simulink model "PubIfDecisionTOS_MDL"  (R2020b)
settings: configuration reference "DspaceConfig" (kept outside this file)
PostLoadFcn:
  | if any(exist('dsrtsu_mdlpostloadfcn', 'file') ~= 0), dsrtsu_mdlpostloadfcn('Execute', bdroot); end
InitFcn:
  | , if any(exist('dsmpb_private', 'file') ~= 0), dsmpb_private('dsmpb_mdlclblib', 'Init', bdroot); end,
undefined symbols (not defined in the file or in its folder): C_TOS_ACCEgoRAxletoFbumplength_m, C_TOS_ACCTargetFront_Flag, C_TOS_AEBJAPedObjDxThre_Val, C_TOS_AEBJAPedObjDyThre_Val, C_TOS_AEBJATargetSize_Val, C_TOS_AEBJAVehObjDxThre_Val, C_TOS_AEBJAVehObjDyThre_Val, C_TOS_AEBJuncPedTargetSize_Val, C_TOS_AEBLatObjDxThre_Val, C_TOS_AEBLatPedDyThre_Val, C_TOS_AEBLatTargetSize_Val, C_TOS_AEBLongTargetInEgoFront_Flag, C_TOS_axAbsGround_Parameter, C_TOS_CameraConfirmedFlag, C_TOS_CNsubjWidth, C_TOS_CurrentLaneCoreMinWidth_Val, C_TOS_CutInProb_Val_Zero, C_TOS_CutOutProb_Val_Zero, C_TOS_D2R_Val, C_TOS_DefaultValueObjectToCenterLine_dy, C_TOS_EgoCarWidth_Val, C_TOS_EgoDxRefPoint_m, C_TOS_EgoRAxletoFbumplength_m, C_TOS_HalfWidthVehicle_Con, C_TOS_HWA_CurrentLaneFlag, C_TOS_HWA_LeftLaneFlag, C_TOS_HWA_MovingDir_Vaild, C_TOS_HWA_MovState_Vaild, C_TOS_HWA_RightLaneFlag, C_TOS_LaneLineCourseErrorFront, C_TOS_LaneLineCourseErrorRear, C_TOS_MotorbikeDefaultWidth_m, C_TOS_NumberOfEffectiveTargets, C_TOS_Obj_Age_Val, C_TOS_Objdx_Constraint_Val, C_TOS_ObjectDefaultWidth_m, C_TOS_ObjInCurrentLane_Val, C_TOS_ObjInCurrentLaneValid, C_TOS_ObjInLeftLaneValid, C_TOS_ObjInRightLaneValid, C_TOS_ObjNotInCurrentLane_Val, C_TOS_ObjNotREElementType, C_TOS_ObjPredictDis_dy_ConstantVal_Zeros, C_TOS_ObjToCenterLine_ConstantVal_Zeros, C_TOS_OFMObjIDInvilad_Val, C_TOS_PIL_LatDisCons_Val_zero, C_TOS_PIL_ObjectCutInFlag_b, C_TOS_PIL_ObjectCutOutFlag_b, C_TOS_PIL_ObjLaneProb_al_Val, C_TOS_PP_ObjFusType_FC_Confirm_b, C_TOS_PP_ObjFusType_FC_FR_Confirm_b, C_TOS_PP_ObjFusType_FR_Confirm_b, C_TOS_RE_80BoolDefault_Val, C_TOS_RE_80Single181Default_Val, C_TOS_RE_80Single255Default_Val, C_TOS_RE_80Uint8Default_Val, C_TOS_RE_D2R, C_TOS_RE_D_180_Val, C_TOS_RE_InvalidObjectID_Val, C_TOS_RE_InvalidTargetChainDir_Val ... (+142)
libraries: simulink x1650, TOS_LIB x361, canfdmsglib x14
(part 63 of 69)

== stateflow chart PubIfDecisionTOS_MDL/TOS_20201112/TOS_2012080320/PP1128/AAT-AdditionalAttributes/RoadEdge/RE_2020_12_07/RoadEdge_V2/RoadEdgeElementFinalJudge/EgoRight_RoadEdgeElementsFinalJudge/RoadEdgeElementFinalJudge ==
  state RoadEdgeElementInJudge [function]
    state RoadEdgeElementTheta1Cal [function]
      state StillTarget13_Theta = Theta_Cal(Target3_Dx,Target1_Dx,Target3_Dy,Target1_Dy,ObjectsSortIndex,ObjectsSortIndex_K1,RE_13TargetTheta_K1) [function]
      state [RE_TooNear2Target_Flag,P_RE_NearTargetThetaOffset] = TargetDisJudge(Target4_Dy,Target3_Dy,Target1_Dy,Target4_Dx,Target3_Dx,Target1_Dx) [function]
      (default) -> (junction 285) : {
          | OFM_Target1_Index = RE_StillObjectSortIndex[i-uint8(3)] - uint8(1) ;
          | OFM_Target3_Index = RE_StillObjectSortIndex[i-uint8(1)] - uint8(1) ;
          | OFM_Target4_Index = RE_StillObjectSortIndex[i] - uint8(1) ;
          | }
      (junction 285) -> (junction 286) : {
          | Target1_Dx = Object_Dx[OFM_Target1_Index] ;
          | Target3_Dx = Object_Dx[OFM_Target3_Index] ;
          | Target4_Dx = Object_Dx[OFM_Target4_Index] ;
          | Target1_Dy = Object_Dy[OFM_Target1_Index] ;
          | Target3_Dy = Object_Dy[OFM_Target3_Index] ;
          | Target4_Dy = Object_Dy[OFM_Target4_Index] ;
          | }
      (junction 286) -> (junction 287) : {
          | ObjectsSortIndex_K1 = RE_StillObjectSortIndex_K1[i];
          | ObjectsSortIndex = RE_StillObjectSortIndex[i];
          | RE_13TargetTheta_K1 = RE_13TargetTheta_ALL[i];
          |
          | StillTarget13_Theta = Theta_Cal(Target3_Dx,Target1_Dx,Target3_Dy,Target1_Dy,ObjectsSortIndex,ObjectsSortIndex_K1,RE_13TargetTheta_K1);
          | StillTarget13_Theta_ALL[i] = StillTarget13_Theta;
          | StillTarget34_13_Theta_ALL[i] = RE_2TargetTheta[i] - StillTarget13_Theta;
          |
          | }
      (junction 287) -> (junction 288) : {
          | [RE_TooNear2Target_Flag,P_RE_NearTargetThetaOffset] = TargetDisJudge(Target4_Dy,Target3_Dy,Target1_Dy,Target4_Dx,Target3_Dx,Target1_Dx);
          | RE_TooNear2Target_Flag_ALL[i] = RE_TooNear2Target_Flag;
          | }
      (junction 288) -> (junction 840)
    state RoadEdgeElement2ndInJudge [function]
      (default) -> (junction 249)
      (junction 249) -> (junction 250) [order 1] : [RE_3TargetTheta[i-uint8(1)] < P_TOS_RE_REE3TargetThetaMax_Val&&...
          | RE_3TargetTheta[i-uint8(1)] > P_TOS_RE_REE3TargetThetaMin_Val]
      (junction 249) -> (junction 257) [order 2] : {
          | RoadEdgeElementFlag[OFM_Target_Index] = false;
          | }
      (junction 250) -> (junction 251)
      (junction 251) -> (junction 252) [order 1] : [Ego_Vxv <= P_TOS_RE_RoadEdgeGroupEgoVxvThre_Val]
      (junction 251) -> (junction 255) [order 2]
      (junction 252) -> (junction 253)
      (junction 253) -> (junction 254) [order 1] : [RE_TooNear2Target_Flag_ALL[i] == false &&...
          | StillTarget34_13_Theta_ALL[i] < P_TOS_RE_LowSpeedREE4TargetThetaMax_Val&&...
          | StillTarget34_13_Theta_ALL[i] > P_TOS_RE_LowSpeedREE4TargetThetaMin_Val]
      (junction 253) -> (junction 854) [order 2]
      (junction 254) -> (junction 261) : {
          | RoadEdgeElementFlag[OFM_Target_Index] = true;
          | }
      (junction 255) -> (junction 256) [order 1] : [RE_TooNear2Target_Flag_ALL[i] == false &&...
          | StillTarget34_13_Theta_ALL[i] < P_TOS_RE_HighSpeedREE4TargetThetaMax_Val&&...
          | StillTarget34_13_Theta_ALL[i] > P_TOS_RE_HighSpeedREE4TargetThetaMin_Val]
      (junction 255) -> (junction 849) [order 2]
      (junction 256) -> (junction 259) : {
          | RoadEdgeElementFlag[OFM_Target_Index] = true;
          | }
      (junction 854) -> (junction 856) [order 1] : [RE_TooNear2Target_Flag_ALL[i] == true &&...
          | StillTarget34_13_Theta_ALL[i] < P_TOS_RE_LowSpeedREE4TargetThetaMax_Val + P_RE_NearTargetThetaOffset &&...
          | StillTarget34_13_Theta_ALL[i] > P_TOS_RE_LowSpeedREE4TargetThetaMin_Val - P_RE_NearTargetThetaOffset]
      (junction 854) -> (junction 260) [order 2] : {
          | RoadEdgeElementFlag[OFM_Target_Index] = false;
          | }
      (junction 856) -> (junction 858) : {
          | RoadEdgeElementFlag[OFM_Target_Index] = true;
          | }
      (junction 849) -> (junction 851) [order 1] : [RE_TooNear2Target_Flag_ALL[i] == true &&...
          | StillTarget34_13_Theta_ALL[i] < P_TOS_RE_HighSpeedREE4TargetThetaMax_Val + P_RE_NearTargetThetaOffset&&...
          | StillTarget34_13_Theta_ALL[i] > P_TOS_RE_HighSpeedREE4TargetThetaMin_Val - P_RE_NearTargetThetaOffset]
      (junction 849) -> (junction 258) [order 2] : {
          | RoadEdgeElementFlag[OFM_Target_Index] = false;
          | }
      (junction 851) -> (junction 846) : {
          | RoadEdgeElementFlag[OFM_Target_Index] = true;
          | }
      (junction 261) -> (junction 858)
      (junction 858) -> (junction 260)
      (junction 258) -> (junction 257)
      (junction 846) -> (junction 258)
      (junction 259) -> (junction 846)
      (junction 260) -> (junction 259)
      (junction 257) -> (junction 262)
    state RoadEdgeElement2ndOutJudge [function]
      (default) -> (junction 864)
      (junction 864) -> (junction 865) [order 1] : [RE_3TargetTheta[i-uint8(1)] < P_TOS_RE_REE3TargetThetaMax_Val&&...
          | RE_3TargetTheta[i-uint8(1)] > P_TOS_RE_REE3TargetThetaMin_Val]
      (junction 864) -> (junction 877) [order 2] : {
          | RoadEdgeElementFlag[OFM_Target_Index] = false;
          | }
      (junction 865) -> (junction 867)
      (junction 867) -> (junction 866) [order 1] : [Ego_Vxv <= P_TOS_RE_RoadEdgeGroupEgoVxvThre_Val]
      (junction 867) -> (junction 868) [order 2]
      (junction 866) -> (junction 873)
      (junction 873) -> (junction 874) [order 1] : [RE_TooNear2Target_Flag_ALL[i] == false &&...
          | StillTarget34_13_Theta_ALL[i] < P_TOS_RE_LowSpeedREE4TargetThetaMaxOut_Val&&...
          | StillTarget34_13_Theta_ALL[i] > P_TOS_RE_LowSpeedREE4TargetThetaMinOut_Val]
      (junction 873) -> (junction 903) [order 2]
      (junction 874) -> (junction 878) : {
          | RoadEdgeElementFlag[OFM_Target_Index] = true;
          | }
      (junction 868) -> (junction 872) [order 1] : [RE_TooNear2Target_Flag_ALL[i] == false &&...
          | StillTarget34_13_Theta_ALL[i] < P_TOS_RE_HighSpeedREE4TargetThetaMaxOut_Val&&...
          | StillTarget34_13_Theta_ALL[i] > P_TOS_RE_HighSpeedREE4TargetThetaMinOut_Val]
      (junction 868) -> (junction 898) [order 2]
      (junction 872) -> (junction 876) : {
          | RoadEdgeElementFlag[OFM_Target_Index] = true;
          | }
      (junction 903) -> (junction 863) [order 1] : [RE_TooNear2Target_Flag_ALL[i] == true &&...
          | StillTarget34_13_Theta_ALL[i] < P_TOS_RE_LowSpeedREE4TargetThetaMaxOut_Val + P_RE_NearTargetThetaOffset &&...
          | StillTarget34_13_Theta_ALL[i] > P_TOS_RE_LowSpeedREE4TargetThetaMinOut_Val - P_RE_NearTargetThetaOffset]
      (junction 903) -> (junction 871) [order 2] : {
          | RoadEdgeElementFlag[OFM_Target_Index] = false;
          | }
      (junction 863) -> (junction 861) : {
          | RoadEdgeElementFlag[OFM_Target_Index] = true;
          | }
      (junction 898) -> (junction 897) [order 1] : [RE_TooNear2Target_Flag_ALL[i] == true &&...
          | StillTarget34_13_Theta_ALL[i] < P_TOS_RE_HighSpeedREE4TargetThetaMaxOut_Val + P_RE_NearTargetThetaOffset&&...
          | StillTarget34_13_Theta_ALL[i] > P_TOS_RE_HighSpeedREE4TargetThetaMinOut_Val - P_RE_NearTargetThetaOffset]
      (junction 898) -> (junction 875) [order 2] : {
          | RoadEdgeElementFlag[OFM_Target_Index] = false;
          | }
      (junction 897) -> (junction 900) : {
          | RoadEdgeElementFlag[OFM_Target_Index] = true;
          | }
      (junction 878) -> (junction 861)
      (junction 861) -> (junction 871)
      (junction 875) -> (junction 877)
      (junction 900) -> (junction 875)
      (junction 876) -> (junction 900)
      (junction 871) -> (junction 876)
      (junction 877) -> (junction 869)
    state RoadEdgeElement3rdInJudge [function]
      (default) -> (junction 300)
      (junction 300) -> (junction 301) [order 1] : [RE_3TargetTheta[i-uint8(2)] < P_TOS_RE_REE3TargetThetaMax_Val&&...
          | RE_3TargetTheta[i-uint8(2)] > P_TOS_RE_REE3TargetThetaMin_Val]
      (junction 300) -> (junction 308) [order 2] : {
          | RoadEdgeElementFlag[OFM_Target_Index] = false;
          | }
      (junction 301) -> (junction 302)
      (junction 302) -> (junction 303) [order 1] : [Ego_Vxv <= P_TOS_RE_RoadEdgeGroupEgoVxvThre_Val]
      (junction 302) -> (junction 304) [order 2]
      (junction 303) -> (junction 306)
      (junction 306) -> (junction 307) [order 1] : [RE_TooNear2Target_Flag_ALL[i] == false &&...
          | (StillTarget34_13_Theta_ALL[i-uint8(1)] < P_TOS_RE_HighSpeedREE4TargetThetaMax_Val&&...
          | StillTarget34_13_Theta_ALL[i-uint8(1)] > P_TOS_RE_HighSpeedREE4TargetThetaMin_Val)&&...
          | (StillTarget34_13_Theta_ALL[i] < P_TOS_RE_LowSpeedREE4TargetThetaMax_Val&&...
          | StillTarget34_13_Theta_ALL[i] > P_TOS_RE_LowSpeedREE4TargetThetaMin_Val)]
      (junction 306) -> (junction 914) [order 2]
      (junction 307) -> (junction 312) : {
          | RoadEdgeElementFlag[OFM_Target_Index] = true;
          | }
      (junction 304) -> (junction 305) [order 1] : [RE_TooNear2Target_Flag_ALL[i] == false &&...
          | (StillTarget34_13_Theta_ALL[i-uint8(1)] < P_TOS_RE_HighSpeedREE4TargetThetaMax_Val&&...
          | StillTarget34_13_Theta_ALL[i-uint8(1)] > P_TOS_RE_HighSpeedREE4TargetThetaMin_Val)&&...
          | (StillTarget34_13_Theta_ALL[i] < P_TOS_RE_HighSpeedREE4TargetThetaMax_Val&&...
          | StillTarget34_13_Theta_ALL[i] > P_TOS_RE_HighSpeedREE4TargetThetaMin_Val)]
      (junction 304) -> (junction 907) [order 2]
      (junction 305) -> (junction 310) : {
          | RoadEdgeElementFlag[OFM_Target_Index] = true;
          | }
      (junction 914) -> (junction 916) [order 1] : [RE_TooNear2Target_Flag_ALL[i] == true &&...
          | (StillTarget34_13_Theta_ALL[i-uint8(1)] < P_TOS_RE_HighSpeedREE4TargetThetaMax_Val + P_RE_NearTargetThetaOffset&&...
          | StillTarget34_13_Theta_ALL[i-uint8(1)] > P_TOS_RE_HighSpeedREE4TargetThetaMin_Val - P_RE_NearTargetThetaOffset)&&...
          | (StillTarget34_13_Theta_ALL[i] < P_TOS_RE_LowSpeedREE4TargetThetaMax_Val + P_RE_NearTargetThetaOffset&&...
          | StillTarget34_13_Theta_ALL[i] > P_TOS_RE_LowSpeedREE4TargetThetaMin_Val - P_RE_NearTargetThetaOffset)]
      (junction 907) -> (junction 909) [order 1] : [RE_TooNear2Target_Flag_ALL[i] == true &&...
          | (StillTarget34_13_Theta_ALL[i-uint8(1)] < P_TOS_RE_HighSpeedREE4TargetThetaMax_Val + P_RE_NearTargetThetaOffset&&...
          | StillTarget34_13_Theta_ALL[i-uint8(1)] > P_TOS_RE_HighSpeedREE4TargetThetaMin_Val - P_RE_NearTargetThetaOffset)&&...
          | (StillTarget34_13_Theta_ALL[i] < P_TOS_RE_HighSpeedREE4TargetThetaMax_Val + P_RE_NearTargetThetaOffset&&...
          | StillTarget34_13_Theta_ALL[i] > P_TOS_RE_HighSpeedREE4TargetThetaMin_Val - P_RE_NearTargetThetaOffset)]
      (junction 914) -> (junction 311) [order 2] : {
          | RoadEdgeElementFlag[OFM_Target_Index] = false;
          | }
      (junction 916) -> (junction 918) : {
          | RoadEdgeElementFlag[OFM_Target_Index] = true;
          | }
      (junction 907) -> (junction 309) [order 2] : {
          | RoadEdgeElementFlag[OFM_Target_Index] = false;
          | }
      (junction 909) -> (junction 911) : {
          | RoadEdgeElementFlag[OFM_Target_Index] = true;
          | }
      (junction 309) -> (junction 308)
      (junction 911) -> (junction 309)
      (junction 310) -> (junction 911)
      (junction 311) -> (junction 310)
      (junction 918) -> (junction 311)
      (junction 312) -> (junction 918)
      (junction 308) -> (junction 313)
    state RoadEdgeElement3rdOutJudge [function]
      (default) -> (junction 924)
      (junction 924) -> (junction 921) [order 1] : [RE_3TargetTheta[i-uint8(2)] < P_TOS_RE_REE3TargetThetaMax_Val&&...
          | RE_3TargetTheta[i-uint8(2)] > P_TOS_RE_REE3TargetThetaMin_Val]
      (junction 924) -> (junction 934) [order 2] : {
          | RoadEdgeElementFlag[OFM_Target_Index] = false;
          | }
      (junction 921) -> (junction 933)
      (junction 933) -> (junction 927) [order 1] : [Ego_Vxv <= P_TOS_RE_RoadEdgeGroupEgoVxvThre_Val]
      (junction 933) -> (junction 925) [order 2]
      (junction 927) -> (junction 928)
      (junction 928) -> (junction 932) [order 1] : [RE_TooNear2Target_Flag_ALL[i] == false &&...
          | (StillTarget34_13_Theta_ALL[i-uint8(1)] < P_TOS_RE_HighSpeedREE4TargetThetaMaxOut_Val&&...
          | StillTarget34_13_Theta_ALL[i-uint8(1)] > P_TOS_RE_HighSpeedREE4TargetThetaMinOut_Val)&&...
          | (StillTarget34_13_Theta_ALL[i] < P_TOS_RE_LowSpeedREE4TargetThetaMaxOut_Val&&...
          | StillTarget34_13_Theta_ALL[i] > P_TOS_RE_LowSpeedREE4TargetThetaMinOut_Val)]
      (junction 928) -> (junction 965) [order 2]
      (junction 932) -> (junction 937) : {
          | RoadEdgeElementFlag[OFM_Target_Index] = true;
          | }
      (junction 925) -> (junction 938) [order 1] : [RE_TooNear2Target_Flag_ALL[i] == false &&...
          | (StillTarget34_13_Theta_ALL[i-uint8(1)] < P_TOS_RE_HighSpeedREE4TargetThetaMaxOut_Val&&...
          | StillTarget34_13_Theta_ALL[i-uint8(1)] > P_TOS_RE_HighSpeedREE4TargetThetaMinOut_Val)&&...
          | (StillTarget34_13_Theta_ALL[i] < P_TOS_RE_HighSpeedREE4TargetThetaMaxOut_Val&&...
          | StillTarget34_13_Theta_ALL[i] > P_TOS_RE_HighSpeedREE4TargetThetaMinOut_Val)]
      (junction 925) -> (junction 956) [order 2]
      (junction 938) -> (junction 929) : {
          | RoadEdgeElementFlag[OFM_Target_Index] = true;
          | }
      (junction 965) -> (junction 957) [order 1] : [RE_TooNear2Target_Flag_ALL[i] == true &&...
          | (StillTarget34_13_Theta_ALL[i-uint8(1)] < P_TOS_RE_HighSpeedREE4TargetThetaMaxOut_Val + P_RE_NearTargetThetaOffset&&...
          | StillTarget34_13_Theta_ALL[i-uint8(1)] > P_TOS_RE_HighSpeedREE4TargetThetaMinOut_Val - P_RE_NearTargetThetaOffset)&&...
          | (StillTarget34_13_Theta_ALL[i] < P_TOS_RE_LowSpeedREE4TargetThetaMaxOut_Val + P_RE_NearTargetThetaOffset&&...
          | StillTarget34_13_Theta_ALL[i] > P_TOS_RE_LowSpeedREE4TargetThetaMinOut_Val - P_RE_NearTargetThetaOffset)]
      (junction 956) -> (junction 962) [order 1] : [RE_TooNear2Target_Flag_ALL[i] == true &&...
          | (StillTarget34_13_Theta_ALL[i-uint8(1)] < P_TOS_RE_HighSpeedREE4TargetThetaMaxOut_Val + P_RE_NearTargetThetaOffset&&...
          | StillTarget34_13_Theta_ALL[i-uint8(1)] > P_TOS_RE_HighSpeedREE4TargetThetaMinOut_Val - P_RE_NearTargetThetaOffset)&&...
          | (StillTarget34_13_Theta_ALL[i] < P_TOS_RE_HighSpeedREE4TargetThetaMaxOut_Val + P_RE_NearTargetThetaOffset&&...
          | StillTarget34_13_Theta_ALL[i] > P_TOS_RE_HighSpeedREE4TargetThetaMinOut_Val - P_RE_NearTargetThetaOffset)]
      (junction 965) -> (junction 940) [order 2] : {
          | RoadEdgeElementFlag[OFM_Target_Index] = false;
          | }
      (junction 957) -> (junction 954) : {
          | RoadEdgeElementFlag[OFM_Target_Index] = true;
          | }
      (junction 956) -> (junction 936) [order 2] : {
          | RoadEdgeElementFlag[OFM_Target_Index] = false;
          | }
      (junction 962) -> (junction 959) : {
          | RoadEdgeElementFlag[OFM_Target_Index] = true;
          | }
      (junction 936) -> (junction 934)
      (junction 959) -> (junction 936)
      (junction 929) -> (junction 959)
      (junction 940) -> (junction 929)
      (junction 954) -> (junction 940)
      (junction 937) -> (junction 954)
      (junction 934) -> (junction 942)
    state RoadEdgeElement1stInJudge [function]
      (default) -> (junction 333)
      (junction 333) -> (junction 334) [order 1] : [RE_3TargetTheta[i] < P_TOS_RE_REE3TargetThetaMax_Val&&...
          | RE_3TargetTheta[i] > P_TOS_RE_REE3TargetThetaMin_Val]
      (junction 333) -> (junction 335) [order 2] : {
          | RoadEdgeElementFlag[OFM_Target_Index] = false;
          | }
      (junction 334) -> (junction 336) : {
          | RoadEdgeElementFlag[OFM_Target_Index_2 ] = true;
          | RoadEdgeElementFlag[OFM_Target_Index_1 ] = true;
          | RoadEdgeElementFlag[OFM_Target_Index] = true;
          | }
      (junction 336) -> (junction 335)
      (junction 335) -> (junction 337)
    (default) -> (junction 344) : {
        | OFM_Target_Index = RE_StillObjectSortIndex[i]-uint8(1) ;
        | OFM_Target_Index_1 = RE_StillObjectSortIndex[i-uint8(1)]-uint8(1) ;
        | OFM_Target_Index_2 = RE_StillObjectSortIndex[i-uint8(2)]-uint8(1) ;
        | }
    (junction 344) -> (junction 345) [order 1] : [EdgeGroupChainElementCount[i] == uint8(3)]
        | %一条边界组链中的第3个元素
    (junction 344) -> (junction 346) [order 2]
    (junction 345) -> (junction 360) : {
        | RoadEdgeElement1stInJudge();
        | }
    (junction 346) -> (junction 246) [order 1] : [EdgeGroupChainElementCount[i] >= uint8(4)]
        | %一条边界组链中的第4个和以后的元素
    (junction 346) -> (junction 282) [order 2] : {
        | RoadEdgeElementFlag[i] = false;
        | }
    (junction 246) -> (junction 281) : {
        | RoadEdgeElementTheta1Cal();
        | }
    (junction 281) -> (junction 247) [order 1] : [EdgeGroupChainElementCount[i] >= uint8(5)]
        | %一条边界组链中的第5个和以后的元素
    (junction 281) -> (junction 643) [order 2]
    (junction 247) -> (junction 636)
    (junction 636) -> (junction 638) [order 1] : [RE_4StepEdgeElementFlag[OFM_Target_Index] == true]
        | %连续四个周期选中为边界元素
    (junction 643) -> (junction 645) [order 1] : [RE_4StepEdgeElementFlag[OFM_Target_Index] == true]
        | %连续四个周期选中为边界元素
    (junction 636) -> (junction 362) [order 2] : {
        | RoadEdgeElement3rdInJudge();
        | }
    (junction 638) -> (junction 640) : {
        | RoadEdgeElement3rdOutJudge();
        | }
    (junction 643) -> (junction 283) [order 2] : {
        | RoadEdgeElement2ndInJudge();
        | }
    (junction 645) -> (junction 647) : {
        | RoadEdgeElement2ndOutJudge();
        | }
    (junction 283) -> (junction 282)
    (junction 647) -> (junction 283)
    (junction 362) -> (junction 647)
    (junction 640) -> (junction 362)
    (junction 360) -> (junction 640)
    (junction 282) -> (junction 480)
  state RoadEdgeElementOFMSort [function]
    (default) -> (junction 489)
    (junction 489) -> (junction 506) [order 1] : [RoadEdgeElementFlag[OFM_Target_Index] == true]
    (junction 506) -> (junction 502) : {
        | RE_EdgeElementType[OFM_Target_Index] = uint8(2);
        | RE_EdgeElementID[OFM_Target_Index] = Object_ID[OFM_Target_Index];
        | }
    (junction 489) -> (junction 495) [order 2] : %donothing
    (junction 502) -> (junction 494) [order 1] : [RoadEdgeElementFlag[OFM_Target_Index_1] == true]
    (junction 502) -> (junction 505) [order 2] : %donothing
    (junction 494) -> (junction 504) : {
        | RE_EdgeElementType[OFM_Target_Index_1] = uint8(2);
        | RE_EdgeElementID[OFM_Target_Index_1] = Object_ID[OFM_Target_Index_1];
        | }
    (junction 504) -> (junction 499) [order 1] : [RoadEdgeElementFlag[OFM_Target_Index_2] == true]
    (junction 499) -> (junction 493) : {
        | RE_EdgeElementType[OFM_Target_Index_2] = uint8(2);
        | RE_EdgeElementID[OFM_Target_Index_2] = Object_ID[OFM_Target_Index_2];
        | }
    (junction 504) -> (junction 492) [order 2] : %donothing
    (junction 505) -> (junction 495)
    (junction 492) -> (junction 505)
    (junction 493) -> (junction 492)
    (junction 495) -> (junction 512)
  state RoadEdgeElementInfo_OFM [function]
    (default) -> (junction 982) : {
        | OFM_Target_Index = RE_StillObjectSortIndex[i]-uint8(1) ;
        | }
    (junction 982) -> (junction 983) : {
        | EdgeGroupChainElementCount_OFM[OFM_Target_Index] = EdgeGroupChainElementCount[i];
        | EdgeGroupChainElementCount_OFM[RE_StillObjectSortIndex[0]-uint8(1)] = EdgeGroupChainElementCount[0];
        | EdgeGroupChainElementCount_OFM[RE_StillObjectSortIndex[1]-uint8(1)] = EdgeGroupChainElementCount[1];
        |
        | StillTarget13_Theta_OFM[OFM_Target_Index] = StillTarget13_Theta;
        | StillTarget34_13_Theta_OFM[OFM_Target_Index] = StillTarget34_13_Theta_ALL[i];
        | StillTarget3Theta_OFM[OFM_Target_Index] = RE_3TargetTheta[i];
        | StillTarget2Theta_OFM[OFM_Target_Index] = RE_2TargetTheta[i];
        |
        |
        | StillTarget2Theta_OFM[RE_StillObjectSortIndex[0]-uint8(1)] = RE_2TargetTheta[0];
        |
        |
        | StillTarget3Theta_OFM[RE_StillObjectSortIndex[1]-uint8(1)] = RE_3TargetTheta[1];
        | StillTarget2Theta_OFM[RE_StillObjectSortIndex[1]-uint8(1)] = RE_2TargetTheta[1];
        | }
    (junction 983) -> (junction 1006)
  (default) -> (junction 35) : {
      | i = uint8(2);
      | RoadEdgeElementFlag = C_TOS_RE_80BoolDefault_Val;
      | RE_EdgeElementType = C_TOS_RE_80Uint8Default_Val;
      | RE_EdgeElementID = C_TOS_RE_80Uint8Default_Val;
      | StillTarget13_Theta = single(181);
      | StillTarget34_13_Theta_ALL = C_TOS_RE_80Single181Default_Val;
      | EdgeGroupChainElementCount_OFM = C_TOS_RE_80Uint8Default_Val;
      |
      | StillTarget2Theta_OFM = C_TOS_RE_80Single181Default_Val;
      | StillTarget3Theta_OFM = C_TOS_RE_80Single181Default_Val;
      | StillTarget34_13_Theta_OFM = C_TOS_RE_80Single181Default_Val;
      | StillTarget13_Theta_OFM = C_TOS_RE_80Single181Default_Val;%观测量
      | }
      | %从第三个目标开始计算判断
  (junction 35) -> (junction 37) [order 1] : [RE_StillObjectSortIndex[i] ~= C_TOS_StillObjSortInvalidIndex_Val &&...
      | i <= uint8(79)]
  (junction 978) -> (junction 35) : {
      | i = i+uint8(1);
      | }
  (junction 35) -> (junction 40) [order 2]
  (junction 37) -> (junction 514) : {
      | RoadEdgeElementInJudge();
      | }
  (junction 514) -> (junction 515) : {
      | RoadEdgeElementOFMSort();
      | }
  (junction 40) -> (junction 43)
  (junction 515) -> (junction 978) : {
      | RoadEdgeElementInfo_OFM();
      | }
  data: Target3_Dx function_input single size=1; Target1_Dx function_input single size=1; Target3_Dy function_input single size=1; Target1_Dy function_input single size=1; StillTarget13_Theta function_output single size=1; ObjectsSortIndex function_input; ObjectsSortIndex_K1 function_input; RE_13TargetTheta_K1 function_input; Target4_Dy function_input single size=1; Target3_Dy function_input single size=1; Target1_Dy function_input single size=1; Target4_Dx function_input single size=1; Target3_Dx function_input single size=1; Target1_Dx function_input single size=1; RE_TooNear2Target_Flag function_output; P_RE_NearTargetThetaOffset function_output; RE_4StepEdgeElementFlag input; C_TOS_StillObjSortInvalidIndex_Val parameter; EdgeGroupChainElementCount input; RE_3TargetTheta input; RE_2TargetTheta input; RE_StillObjectSortIndex input; RE_StillObjectSortIndex_K1 input; Ego_Vxv input; Object_Dx input; Object_Dy input; P_TOS_RE_REE3TargetThetaMax_Val parameter; P_TOS_RE_REE3TargetThetaMin_Val parameter; P_TOS_RE_HighSpeedREE4TargetThetaMax_Val parameter; P_TOS_RE_HighSpeedREE4TargetThetaMin_Val parameter; P_TOS_RE_LowSpeedREE4TargetThetaMax_Val parameter; P_TOS_RE_LowSpeedREE4TargetThetaMin_Val parameter; P_TOS_RE_RoadEdgeGroupEgoVxvThre_Val parameter; OFM_Target1_Index local uint8 size=1; OFM_Target3_Index local uint8 size=1; Target1_Dx local single size=1; Target1_Dy local single size=1; Target3_Dx local single size=1; Target3_Dy local single size=1; i local uint8 size=1; RoadEdgeElementFlag output boolean size=80; Object_ID input; RE_EdgeElementType output uint8 size=80; OFM_Target_Index local uint8 size=1; C_TOS_RE_80BoolDefault_Val parameter; C_TOS_RE_80Single181Default_Val parameter; C_TOS_RE_80Uint8Default_Val parameter; StillTarget34_13_Theta_ALL output single size=80; StillTarget13_Theta local single size=1; RE_EdgeElementID output uint8 size=80; P_TOS_RE_HighSpeedREE4TargetThetaMaxOut_Val parameter; P_TOS_RE_HighSpeedREE4TargetThetaMinOut_Val parameter; P_TOS_RE_LowSpeedREE4TargetThetaMaxOut_Val parameter; P_TOS_RE_LowSpeedREE4TargetThetaMinOut_Val parameter; OFM_Target_Index_1 local uint8; OFM_Target_Index_2 local uint8; RE_13TargetTheta_ALL input; StillTarget13_Theta_ALL output single size=80; ObjectsSortIndex local uint8; ObjectsSortIndex_K1 local uint8; RE_13TargetTheta_K1 local single; StillTarget13_Theta_OFM output single size=80; StillTarget34_13_Theta_OFM output single size=80; StillTarget3Theta_OFM output single size=80; StillTarget2Theta_OFM output single size=80; EdgeGroupChainElementCount_OFM output uint8 size=80; P_RE_NearTargetThetaOffset local single; OFM_Target4_Index local uint8 size=1; RE_TooNear2Target_Flag local boolean size=1; RE_TooNear2Target_Flag_ALL local boolean size=80; Target4_Dx local single size=1; Target4_Dy local single size=1

== stateflow chart PubIfDecisionTOS_MDL/TOS_20201112/TOS_2012080320/TOS/ACC/TOS_ACCCurrentLane/ACCTargetInfor/TOS_ACCP0TargetInfor ==
  (default) -> (junction 1)
  (junction 1) -> (junction 3) [order 1] : [TOS_ACCPO0TargetIndex ~= uint8(0)]
  (junction 1) -> (junction 7) [order 2] : {TOS_ACCPO0TargetInfo.IDP0= uint8(0);
      | TOS_ACCPO0TargetInfo.dxP0=single(255);
      | TOS_ACCPO0TargetInfo.vxRelP0= single(0);
      | TOS_ACCPO0TargetInfo.ACCTgtObjVy=single(0);
      | TOS_ACCPO0TargetInfo.axAbsGroundP0=single(0);
      | TOS_ACCPO0TargetInfo.rangeP0=single(0);
      | TOS_ACCPO0TargetInfo.targetExistP0= boolean(0);
      | TOS_ACCPO0TargetInfo.fu_typeP0= uint8(0);
      | TOS_ACCPO0TargetInfo.ObjMovingStateP0= uint8(0);
      | TOS_ACCPO0TargetInfo.Object_Orientation= uint8(0);
      | TOS_ACCPO0TargetInfo.ObjTypeP0= uint8(0);
      | TOS_ACCPO0TargetInfo.ObjDYP0=single(255);
      | TOS_ACCPO0TargetInfo.ACCTgtObjObstcl=single(0);
      | TOS_ACCPO0TargetInfo.ACCTgtObjAy=single(0);
      | TOS_ACCPO0TargetInfo.ACCTgtObjCntAlive=single(0);
      | TOS_ACCPO0TargetInfo.ACCTgtObjExist=single(0);
      | TOS_ACCPO0TargetInfo.P0HeadingAngle=single(0);
      | TOS_ACCPO0TargetInfo.P0CutInflg= boolean(0);
      | }
  (junction 3) -> (junction 5) : {
      | TOS_ACCPO0TargetInfo.IDP0                      =OFM_SignalVerification.Object_ID[TOS_ACCPO0TargetIndex- uint8(1)];
      | TOS_ACCPO0TargetInfo.dxP0                      =OFM_SignalVerification.Object_DX[TOS_ACCPO0TargetIndex-uint8(1)];
      | TOS_ACCPO0TargetInfo.vxRelP0                 =OFM_SignalVerification.Object_VX[TOS_ACCPO0TargetIndex-uint8(1)];
      | TOS_ACCPO0TargetInfo.ACCTgtObjVy        =OFM_SignalVerification.Object_VY[TOS_ACCPO0TargetIndex-uint8(1)];
      | TOS_ACCPO0TargetInfo.axAbsGroundP0    =TOS_AddAttributes.PP_axAbsGround[TOS_ACCPO0TargetIndex-uint8(1)];
      | TOS_ACCPO0TargetInfo.rangeP0                 =TOS_AddAttributes.PP_ObjToEgoCarFrontbump[TOS_ACCPO0TargetIndex-uint8(1)];
      | TOS_ACCPO0TargetInfo.targetExistP0         =boolean(1);
      | TOS_ACCPO0TargetInfo.fu_typeP0              =OFM_SignalVerification.Object_Fus_Type[TOS_ACCPO0TargetIndex-uint8(1)];
      | TOS_ACCPO0TargetInfo.ObjMovingStateP0 =TOS_AddAttributes.PP_MovingStateSignalProcessing[TOS_ACCPO0TargetIndex-uint8(1)];
      | TOS_ACCPO0TargetInfo.Object_Orientation =TOS_AddAttributes.PP_ObjMovingDirSignalProcessing[TOS_ACCPO0TargetIndex-uint8(1)];
      | TOS_ACCPO0TargetInfo.ObjTypeP0              =OFM_SignalVerification.Object_Type[TOS_ACCPO0TargetIndex-uint8(1)];
      | TOS_ACCPO0TargetInfo.ObjDYP0                 =OFM_SignalVerification.Object_DY[TOS_ACCPO0TargetIndex-uint8(1)];
      | TOS_ACCPO0TargetInfo.ACCTgtObjObstcl    =OFM_SignalVerification.Object_ObstacleProb[TOS_ACCPO0TargetIndex-uint8(1)];
      | TOS_ACCPO0TargetInfo.ACCTgtObjAy          =OFM_SignalVerification.Object_AY[TOS_ACCPO0TargetIndex-uint8(1)];
      | TOS_ACCPO0TargetInfo.ACCTgtObjCntAlive =OFM_SignalVerification.Object_Age[TOS_ACCPO0TargetIndex-uint8(1)];
      | TOS_ACCPO0TargetInfo.ACCTgtObjExist       =OFM_SignalVerification.Object_ExistProb[TOS_ACCPO0TargetIndex-uint8(1)];
      | TOS_ACCPO0TargetInfo.P0HeadingAngle      =OFM_SignalVerification.Object_HeadingAngle[TOS_ACCPO0TargetIndex-uint8(1)];
      | TOS_ACCPO0TargetInfo.P0CutInflg                =TOS_ProbInLaneCalculat.PIL_CutinFlag[TOS_ACCPO0TargetIndex-uint8(1)];
      | }
  (junction 5) -> (junction 7)
  (junction 7) -> (junction 11)
  data: OFM_SignalVerification input Bus: OFM_OBJ_BUS; TOS_AddAttributes input Bus: TOS_AddAttributes_BUS; TOS_ProbInLaneCalculat input Bus: PIL_ProbInLaneCalculat_BUS; TOS_ACCPO0TargetIndex input uint8; TOS_ACCPO0TargetInfo output Bus: TOS_ACCP0_BUS =0

== stateflow chart PubIfDecisionTOS_MDL/TOS_20201112/TOS_2012080320/TOS/ACC/TOS_ACCCurrentLane/ACCTargetInfor/TOS_ACCP1TargetInfor ==
  (default) -> (junction 1)
  (junction 1) -> (junction 3) [order 1] : [TOS_ACCPO1TargetIndex ~= uint8(0)&&...
      | IDP0 ~= uint8(0)]
  (junction 1) -> (junction 7) [order 2] : {
      | TOS_ACCPO1TargetInfo.IDP1= uint8(0);
      | TOS_ACCPO1TargetInfo.dxP1=single(255);
      | TOS_ACCPO1TargetInfo.vxRelP1=single(0);
      | TOS_ACCPO1TargetInfo.axAbsGroundP1=single(0);
      | TOS_ACCPO1TargetInfo.rangeP1=single(0);
      | TOS_ACCPO1TargetInfo.targetExistP1= boolean(1);
      | TOS_ACCPO1TargetInfo.fu_typeP1= uint8(0);
      | TOS_ACCPO1TargetInfo.ObjMovingStateP1= uint8(0);
      | TOS_ACCPO1TargetInfo.ObjTypeP1= uint8(0);
      | TOS_ACCPO1TargetInfo.ObjDYP1= single(255);
      | TOS_ACCPO1TargetInfo.P1HeadingAngle=single(0);
      | }
  (junction 3) -> (junction 5) : {
      | TOS_ACCPO1TargetInfo.IDP1                         = OFM_SignalVerification.Object_ID[TOS_ACCPO1TargetIndex-uint8(1)];
      | TOS_ACCPO1TargetInfo.dxP1                         = OFM_SignalVerification.Object_DX[TOS_ACCPO1TargetIndex-uint8(1)];
      | TOS_ACCPO1TargetInfo.vxRelP1                    = OFM_SignalVerification.Object_VX[TOS_ACCPO1TargetIndex-uint8(1)];
      | TOS_ACCPO1TargetInfo.axAbsGroundP1       = TOS_AddAttributes.PP_axAbsGround[TOS_ACCPO1TargetIndex-uint8(1)];
      | TOS_ACCPO1TargetInfo.rangeP1                    = TOS_AddAttributes.PP_ObjToEgoCarFrontbump[TOS_ACCPO1TargetIndex-uint8(1)];
      | TOS_ACCPO1TargetInfo.targetExistP1            = boolean(1);
      | TOS_ACCPO1TargetInfo.fu_typeP1                 = OFM_SignalVerification.Object_Fus_Type[TOS_ACCPO1TargetIndex-uint8(1)];
      | TOS_ACCPO1TargetInfo.ObjMovingStateP1   = TOS_AddAttributes.PP_MovingStateSignalProcessing[TOS_ACCPO1TargetIndex-uint8(1)];
      | TOS_ACCPO1TargetInfo.ObjTypeP1               = OFM_SignalVerification.Object_Type[TOS_ACCPO1TargetIndex-uint8(1)];
      | TOS_ACCPO1TargetInfo.ObjDYP1                  = OFM_SignalVerification.Object_DY[TOS_ACCPO1TargetIndex-uint8(1)];
      | TOS_ACCPO1TargetInfo.P1HeadingAngle      = OFM_SignalVerification.Object_HeadingAngle[TOS_ACCPO1TargetIndex-uint8(1)];
      | }
  (junction 5) -> (junction 7)
  (junction 7) -> (junction 11)
  data: IDP0 input; OFM_SignalVerification input Bus: OFM_OBJ_BUS; TOS_AddAttributes input Bus: TOS_AddAttributes_BUS; TOS_ACCPO1TargetIndex input uint8; TOS_ACCPO1TargetInfo output Bus: TOS_ACCP1_BUS

== stateflow chart PubIfDecisionTOS_MDL/TOS_20201112/TOS_2012080320/TOS/ACC/TOS_ACCCurrentLane/ACC_CurrentLane_Target/TOS_ACC_P0/ACC_P0_Targe/ACC_P0_Targe/TOS_ACC_FusionTypeConfirm/Subsystem1/TOS_ObjMovStateCfmFlow1 ==
  note: TOS_ObjMovStateCfm Coding:
      | 0: Object default moving state
      | 1：Object had been moving
      | 2: Object is moving
  (default) -> (junction 1)
  (junction 1) -> (junction 3) [order 1] : [Target_ID_K1 ~=C_TOS_OFMObjIDInvilad_Val&&...
      | Target_ID_K2 ~= C_TOS_OFMObjIDInvilad_Val]
  (junction 1) -> (junction 38) [order 2] : {
      |   TOS_ObjMovStateCfm = uint8(0);
      | }
  (junction 3) -> (junction 5)
  (junction 5) -> (junction 7) [order 1] : [Target_ID_K1 ==Target_ID_K2]
  (junction 5) -> (junction 35) [order 2] : {
      |   TOS_ObjMovStateCfm =uint8(0);
      | }
  (junction 7) -> (junction 9)
  (junction 9) -> (junction 11) [order 1] : [ObjectID ==Target_ID_K1]
  (junction 9) -> (junction 29) [order 2] : {
      |   TOS_ObjMovStateCfm = uint8(0);
      | }
  (junction 11) -> (junction 13)
  (junction 13) -> (junction 15) [order 1] : [(Target_MovState_K2 == ObjectMovingState_E.Moving||...
      | Target_MovState_K2 == ObjectMovingState_E.Stopped)&&...
      | (Target_MovState_K1 == ObjectMovingState_E.Moving||...
      | Target_MovState_K1 == ObjectMovingState_E.Stopped)||...
      |   TOS_ObjMovStateCfm == uint8(1)]
  (junction 13) -> (junction 52) [order 2]
  (junction 15) -> (junction 58) : {
      |   TOS_ObjMovStateCfm = uint8(1);
      | }
  (junction 52) -> (junction 23) [order 1] : [ObjMovState == OFM_OBJ_MOVINGSTATE_E.STOPPED||...
      | ObjMovState == OFM_OBJ_MOVINGSTATE_E.MOVING]
  (junction 52) -> (junction 27) [order 2] : {
      |   TOS_ObjMovStateCfm = uint8(0);
      | }
  (junction 23) -> (junction 54) : {
      |   TOS_ObjMovStateCfm = uint8(2);
      | }
  (junction 35) -> (junction 38)
  (junction 29) -> (junction 35)
  (junction 27) -> (junction 29)
  (junction 54) -> (junction 27)
  (junction 58) -> (junction 54)
  (junction 38) -> (junction 41)
  data: Target_ID_K1 input uint8; Target_ID_K2 input uint8; Target_MovState_K1 input Enum: ObjectMovingState_E; Target_MovState_K2 input Enum: ObjectMovingState_E; ObjMovState input Enum: OFM_OBJ_MOVINGSTATE_E; ObjectID input uint8; TOS_ObjMovStateCfm output uint8; C_TOS_OFMObjIDInvilad_Val parameter uint8

== stateflow chart PubIfDecisionTOS_MDL/TOS_20201112/TOS_2012080320/TOS/ACC/TOS_ACCCurrentLane/ACC_CurrentLane_Target/TOS_ACC_P0/ACC_P0_Targe/ACC_P0_Targe/TOS_ACC_ObjTypeConfirm/Subsystem/TOS_ObjMovStateCfmFlow1 ==
  note: TOS_ObjMovStateCfm Coding:
      | 0: Object default moving state
      | 1：Object had been moving
      | 2: Object is moving
  (default) -> (junction 1)
  (junction 1) -> (junction 3) [order 1] : [ACC_TargetP0_ID_K1 ~=C_TOS_OFMObjIDInvilad_Val&&...
      | ACC_TargetP0_ID_K2 ~= C_TOS_OFMObjIDInvilad_Val]
  (junction 1) -> (junction 38) [order 2] : {
      |   TOS_ObjMovStateCfm = uint8(0);
      | }
  (junction 3) -> (junction 5)
  (junction 5) -> (junction 7) [order 1] : [ACC_TargetP0_ID_K1 ==ACC_TargetP0_ID_K2]
  (junction 5) -> (junction 35) [order 2] : {
      |   TOS_ObjMovStateCfm =uint8(0);
      | }
  (junction 7) -> (junction 9)
  (junction 9) -> (junction 11) [order 1] : [ObjectID ==ACC_TargetP0_ID_K1]
  (junction 9) -> (junction 29) [order 2] : {
      |   TOS_ObjMovStateCfm = uint8(0);
      | }
  (junction 11) -> (junction 13)
  (junction 13) -> (junction 15) [order 1] : [(ACC_TargetP0_MovState_K2 == ObjectMovingState_E.Moving||...
      | ACC_TargetP0_MovState_K2 == ObjectMovingState_E.Stopped)&&...
      | (ACC_TargetP0_MovState_K1 == ObjectMovingState_E.Moving||...
      | ACC_TargetP0_MovState_K1 == ObjectMovingState_E.Stopped)||...
      |   TOS_ObjMovStateCfm == uint8(1)]
  (junction 13) -> (junction 52) [order 2]
  (junction 15) -> (junction 58) : {
      |   TOS_ObjMovStateCfm = uint8(1);
      | }
  (junction 52) -> (junction 23) [order 1] : [ObjMovState == OFM_OBJ_MOVINGSTATE_E.STOPPED||...
      | ObjMovState == OFM_OBJ_MOVINGSTATE_E.MOVING]
  (junction 52) -> (junction 27) [order 2] : {
      |   TOS_ObjMovStateCfm = uint8(0);
      | }
  (junction 23) -> (junction 54) : {
      |   TOS_ObjMovStateCfm = uint8(2);
      | }
  (junction 35) -> (junction 38)
  (junction 29) -> (junction 35)
  (junction 27) -> (junction 29)
  (junction 54) -> (junction 27)
  (junction 58) -> (junction 54)
  (junction 38) -> (junction 41)
  data: ACC_TargetP0_ID_K1 input uint8; ACC_TargetP0_ID_K2 input uint8; ACC_TargetP0_MovState_K1 input Enum: ObjectMovingState_E; ACC_TargetP0_MovState_K2 input Enum: ObjectMovingState_E; ObjMovState input Enum: OFM_OBJ_MOVINGSTATE_E; ObjectID input uint8; TOS_ObjMovStateCfm output uint8; C_TOS_OFMObjIDInvilad_Val parameter uint8

== stateflow chart PubIfDecisionTOS_MDL/TOS_20201112/TOS_2012080320/TOS/ACC/TOS_ACCCurrentLane/ACC_CurrentLane_Target/TOS_ACC_P0/ACC_P0_Targe/ACC_P0_Targe/TOS_ACC_TargetMovingDirConfirm/Subsystem/TOS_ObjMovStateCfmFlow ==
  note: TOS_ObjMovStateCfm Coding:
      | 0: Object default moving state
      | 1：Object had been moving
      | 2: Object had been Stopped
  (default) -> (junction 1)
  (junction 1) -> (junction 3) [order 1] : [Target_ID_K1 ~=C_TOS_OFMObjIDInvilad_Val&&...
      | Target_ID_K2 ~= C_TOS_OFMObjIDInvilad_Val]
  (junction 1) -> (junction 38) [order 2] : {
      |   TOS_ObjMovStateCfm = uint8(0);
      | }
  (junction 3) -> (junction 5)
  (junction 5) -> (junction 7) [order 1] : [Target_ID_K1 ==Target_ID_K2]
  (junction 5) -> (junction 35) [order 2] : {
      |   TOS_ObjMovStateCfm =uint8(0);
      | }
  (junction 7) -> (junction 9)
  (junction 9) -> (junction 11) [order 1] : [ObjectID ==Target_ID_K1]
  (junction 9) -> (junction 29) [order 2] : {
      |   TOS_ObjMovStateCfm = uint8(0);
      | }
  (junction 11) -> (junction 13)
  (junction 13) -> (junction 15) [order 1] : [Target_MovState_K2 == ObjectMovingState_E.Moving&&...
      | Target_MovState_K1 == ObjectMovingState_E.Moving||...
      |   TOS_ObjMovStateCfm == uint8(1)]
  (junction 13) -> (junction 52) [order 2]
  (junction 15) -> (junction 58) : {
      |   TOS_ObjMovStateCfm = uint8(1);
      | }
  (junction 52) -> (junction 23) [order 1] : [Target_MovState_K2 == ObjectMovingState_E.Stopped&&...
      | Target_MovState_K1 == ObjectMovingState_E.Stopped||...
      |   TOS_ObjMovStateCfm == uint8(2)]
  (junction 52) -> (junction 27) [order 2] : {
      |   TOS_ObjMovStateCfm = uint8(0);
      | }
  (junction 23) -> (junction 54) : {
      |   TOS_ObjMovStateCfm = uint8(2);
      | }
  (junction 35) -> (junction 38)
  (junction 29) -> (junction 35)
  (junction 27) -> (junction 29)
  (junction 54) -> (junction 27)
  (junction 58) -> (junction 54)
  (junction 38) -> (junction 41)
  data: Target_ID_K1 input uint8; Target_ID_K2 input uint8; Target_MovState_K1 input Enum: ObjectMovingState_E; Target_MovState_K2 input Enum: ObjectMovingState_E; ObjMovState input Enum: OFM_OBJ_MOVINGSTATE_E; ObjectID input uint8; TOS_ObjMovStateCfm output uint8; C_TOS_OFMObjIDInvilad_Val parameter uint8

== stateflow chart PubIfDecisionTOS_MDL/TOS_20201112/TOS_2012080320/TOS/ACC/TOS_ACCCurrentLane/ACC_CurrentLane_Target/TOS_ACC_P1/ACC_P1_Targe/ACC_P1_Targe/TOS_ACC_FusionTypeConfirm/Subsystem1/TOS_ObjMovStateCfmFlow1 ==
  note: TOS_ObjMovStateCfm Coding:
      | 0: Object default moving state
      | 1：Object had been moving
      | 2: Object is moving
  (default) -> (junction 1)
  (junction 1) -> (junction 3) [order 1] : [Target_ID_K1 ~=C_TOS_OFMObjIDInvilad_Val&&...
      | Target_ID_K2 ~= C_TOS_OFMObjIDInvilad_Val]
  (junction 1) -> (junction 38) [order 2] : {
      |   TOS_ObjMovStateCfm = uint8(0);
      | }
  (junction 3) -> (junction 5)
  (junction 5) -> (junction 7) [order 1] : [Target_ID_K1 ==Target_ID_K2]
  (junction 5) -> (junction 35) [order 2] : {
      |   TOS_ObjMovStateCfm =uint8(0);
      | }
  (junction 7) -> (junction 9)
  (junction 9) -> (junction 11) [order 1] : [ObjectID ==Target_ID_K1]
  (junction 9) -> (junction 29) [order 2] : {
      |   TOS_ObjMovStateCfm = uint8(0);
      | }
  (junction 11) -> (junction 13)
  (junction 13) -> (junction 15) [order 1] : [(Target_MovState_K2 == ObjectMovingState_E.Moving||...
      | Target_MovState_K2 == ObjectMovingState_E.Stopped)&&...
      | (Target_MovState_K1 == ObjectMovingState_E.Moving||...
      | Target_MovState_K1 == ObjectMovingState_E.Stopped)||...
      |   TOS_ObjMovStateCfm == uint8(1)]
  (junction 13) -> (junction 52) [order 2]
  (junction 15) -> (junction 58) : {
      |   TOS_ObjMovStateCfm = uint8(1);
      | }
  (junction 52) -> (junction 23) [order 1] : [ObjMovState == OFM_OBJ_MOVINGSTATE_E.STOPPED||...
      | ObjMovState == OFM_OBJ_MOVINGSTATE_E.MOVING]
  (junction 52) -> (junction 27) [order 2] : {
      |   TOS_ObjMovStateCfm = uint8(0);
      | }
  (junction 23) -> (junction 54) : {
      |   TOS_ObjMovStateCfm = uint8(2);
      | }
  (junction 35) -> (junction 38)
  (junction 29) -> (junction 35)
  (junction 27) -> (junction 29)
  (junction 54) -> (junction 27)
  (junction 58) -> (junction 54)
  (junction 38) -> (junction 41)
  data: Target_ID_K1 input uint8; Target_ID_K2 input uint8; Target_MovState_K1 input Enum: ObjectMovingState_E; Target_MovState_K2 input Enum: ObjectMovingState_E; ObjMovState input Enum: OFM_OBJ_MOVINGSTATE_E; ObjectID input uint8; TOS_ObjMovStateCfm output uint8; C_TOS_OFMObjIDInvilad_Val parameter uint8

== stateflow chart PubIfDecisionTOS_MDL/TOS_20201112/TOS_2012080320/TOS/ACC/TOS_ACCCurrentLane/ACC_CurrentLane_Target/TOS_ACC_P1/ACC_P1_Targe/ACC_P1_Targe/TOS_ACC_ObjTypeConfirm/Subsystem/TOS_ObjMovStateCfmFlow1 ==
  note: TOS_ObjMovStateCfm Coding:
      | 0: Object default moving state
      | 1：Object had been moving
      | 2: Object is moving
  (default) -> (junction 1)
  (junction 1) -> (junction 3) [order 1] : [ACC_TargetP0_ID_K1 ~=C_TOS_OFMObjIDInvilad_Val&&...
      | ACC_TargetP0_ID_K2 ~= C_TOS_OFMObjIDInvilad_Val]
  (junction 1) -> (junction 38) [order 2] : {
      |   TOS_ObjMovStateCfm = uint8(0);
      | }
  (junction 3) -> (junction 5)
  (junction 5) -> (junction 7) [order 1] : [ACC_TargetP0_ID_K1 ==ACC_TargetP0_ID_K2]
  (junction 5) -> (junction 35) [order 2] : {
      |   TOS_ObjMovStateCfm =uint8(0);
      | }
  (junction 7) -> (junction 9)
  (junction 9) -> (junction 11) [order 1] : [ObjectID ==ACC_TargetP0_ID_K1]
  (junction 9) -> (junction 29) [order 2] : {
      |   TOS_ObjMovStateCfm = uint8(0);
      | }
  (junction 11) -> (junction 13)
  (junction 13) -> (junction 15) [order 1] : [(ACC_TargetP0_MovState_K2 == ObjectMovingState_E.Moving||...
      | ACC_TargetP0_MovState_K2 == ObjectMovingState_E.Stopped)&&...
      | (ACC_TargetP0_MovState_K1 == ObjectMovingState_E.Moving||...
      | ACC_TargetP0_MovState_K1 == ObjectMovingState_E.Stopped)||...
      |   TOS_ObjMovStateCfm == uint8(1)]
  (junction 13) -> (junction 52) [order 2]
  (junction 15) -> (junction 58) : {
      |   TOS_ObjMovStateCfm = uint8(1);
      | }
  (junction 52) -> (junction 23) [order 1] : [ObjMovState == OFM_OBJ_MOVINGSTATE_E.STOPPED||...
      | ObjMovState == OFM_OBJ_MOVINGSTATE_E.MOVING]
  (junction 52) -> (junction 27) [order 2] : {
      |   TOS_ObjMovStateCfm = uint8(0);
      | }
  (junction 23) -> (junction 54) : {
      |   TOS_ObjMovStateCfm = uint8(2);
      | }
  (junction 35) -> (junction 38)
  (junction 29) -> (junction 35)
  (junction 27) -> (junction 29)
  (junction 54) -> (junction 27)
  (junction 58) -> (junction 54)
  (junction 38) -> (junction 41)
  data: ACC_TargetP0_ID_K1 input uint8; ACC_TargetP0_ID_K2 input uint8; ACC_TargetP0_MovState_K1 input Enum: ObjectMovingState_E; ACC_TargetP0_MovState_K2 input Enum: ObjectMovingState_E; ObjMovState input Enum: OFM_OBJ_MOVINGSTATE_E; ObjectID input uint8; TOS_ObjMovStateCfm output uint8; C_TOS_OFMObjIDInvilad_Val parameter uint8

== stateflow chart PubIfDecisionTOS_MDL/TOS_20201112/TOS_2012080320/TOS/ACC/TOS_ACCCurrentLane/ACC_CurrentLane_Target/TOS_ACC_P1/ACC_P1_Targe/ACC_P1_Targe/TOS_ACC_TargetMovingDirConfirm/Subsystem/TOS_ObjMovStateCfmFlow ==
  note: TOS_ObjMovStateCfm Coding:
      | 0: Object default moving state
      | 1：Object had been moving
      | 2: Object had been Stopped
  (default) -> (junction 1)
  (junction 1) -> (junction 3) [order 1] : [Target_ID_K1 ~=C_TOS_OFMObjIDInvilad_Val&&...
      | Target_ID_K2 ~= C_TOS_OFMObjIDInvilad_Val]
  (junction 1) -> (junction 38) [order 2] : {
      |   TOS_ObjMovStateCfm = uint8(0);
      | }
  (junction 3) -> (junction 5)
  (junction 5) -> (junction 7) [order 1] : [Target_ID_K1 ==Target_ID_K2]
  (junction 5) -> (junction 35) [order 2] : {
      |   TOS_ObjMovStateCfm =uint8(0);
      | }
  (junction 7) -> (junction 9)
  (junction 9) -> (junction 11) [order 1] : [ObjectID ==Target_ID_K1]
  (junction 9) -> (junction 29) [order 2] : {
      |   TOS_ObjMovStateCfm = uint8(0);
      | }
  (junction 11) -> (junction 13)
  (junction 13) -> (junction 15) [order 1] : [Target_MovState_K2 == ObjectMovingState_E.Moving&&...
      | Target_MovState_K1 == ObjectMovingState_E.Moving||...
      |   TOS_ObjMovStateCfm == uint8(1)]
  (junction 13) -> (junction 52) [order 2]
  (junction 15) -> (junction 58) : {
      |   TOS_ObjMovStateCfm = uint8(1);
      | }
  (junction 52) -> (junction 23) [order 1] : [Target_MovState_K2 == ObjectMovingState_E.Stopped&&...
      | Target_MovState_K1 == ObjectMovingState_E.Stopped||...
      |   TOS_ObjMovStateCfm == uint8(2)]
  (junction 52) -> (junction 27) [order 2] : {
      |   TOS_ObjMovStateCfm = uint8(0);
      | }
  (junction 23) -> (junction 54) : {
      |   TOS_ObjMovStateCfm = uint8(2);
      | }
  (junction 35) -> (junction 38)
  (junction 29) -> (junction 35)
  (junction 27) -> (junction 29)
  (junction 54) -> (junction 27)
  (junction 58) -> (junction 54)
  (junction 38) -> (junction 41)
  data: Target_ID_K1 input uint8; Target_ID_K2 input uint8; Target_MovState_K1 input Enum: ObjectMovingState_E; Target_MovState_K2 input Enum: ObjectMovingState_E; ObjMovState input Enum: OFM_OBJ_MOVINGSTATE_E; ObjectID input uint8; TOS_ObjMovStateCfm output uint8; C_TOS_OFMObjIDInvilad_Val parameter uint8

== stateflow chart PubIfDecisionTOS_MDL/TOS_20201112/TOS_2012080320/TOS/ACC/TOS_ACCCurrentLane/ACC_Object_PreConfirm/ACC_P0_P1_Object_TargPreConfirm/ACC_P0_P1_Object_TargPreConfirm/Subsystem3/Chart ==
  (default) -> (junction 1)
  (junction 1) -> (junction 3) [order 1] : [(FR_Confirm == C_TOS_PP_ObjFusType_FR_Confirm_b)&&...
      | ((Obj_MovingState == OFM_OBJ_MOVINGSTATE_E.STATIONARY)||...
      | (Obj_MovingState == OFM_OBJ_MOVINGSTATE_E.INVALID)||...
      | (Obj_MovingState == OFM_OBJ_MOVINGSTATE_E.UNKNOWN))]
  (junction 1) -> (junction 20) [order 2] : {
      |   ObjectisFence_Flag =false;
      | }
  (junction 3) -> (junction 5)
  (junction 5) -> (junction 35) [order 1] : [Object_ObstacleProb < single(0.85)]
  (junction 5) -> (junction 17) [order 2] : {
      |   ObjectisFence_Flag =false;
      | }
  (junction 35) -> (junction 37)
  (junction 37) -> (junction 39) [order 1] : [abs(Object_DY) < single(1.45) ]
  (junction 37) -> (junction 41) [order 2] : {
      |   ObjectisFence_Flag = true;
      | }
  (junction 39) -> (junction 15) : {
      |   ObjectisFence_Flag = false;
      | }
  (junction 17) -> (junction 20)
  (junction 41) -> (junction 17)
  (junction 15) -> (junction 41)
  (junction 20) -> (junction 23)
  data: FR_Confirm input boolean; Obj_MovingState input Enum: OFM_OBJ_MOVINGSTATE_E; ObjectisFence_Flag output boolean; Object_ObstacleProb input single; Object_DY input single; C_TOS_PP_ObjFusType_FR_Confirm_b parameter

== matlab function PubIfDecisionTOS_MDL/TOS_20201112/TOS_2012080320/TOS/ACC/TOS_ACCCurrentLane/MATLAB Function1 ==
  data: Object_Dx input; Object_ID input; Dx1stNearestObjIndex output; Dx2edNearestObjIndex output; ConditionJudge input; TargetFusionTypeFlag input; Object_Num input; Dx1stNearestObjID output; Dx2edNearestObjID output

%%%%ObjDisIndex按Dx从小到大的总排序
%%%%%%%%ObjectID按Dx从小到大的总排序
function [Dx1stNearestObjIndex,Dx2edNearestObjIndex,Dx1stNearestObjID,Dx2edNearestObjID]   = MinMax(Object_Dx,Object_ID,ConditionJudge,TargetFusionTypeFlag,Object_Num)
Dx = Object_Dx;
ID = Object_ID;
for i=int32(1):int32(Object_Num)
    
    if (ID(i) == uint8(0))||(ConditionJudge(i) == false)||(Dx(i) < single(0))||(TargetFusionTypeFlag(i) == false)%%%%%本车道/前方/非0目标
       Dx(i) = single(255);
    end
end

[MinDx1st,MinIndex1st] = min(Dx);
if (MinDx1st > single(250))
   Dx1stNearestObjIndex = uint8(0);
   Dx1stNearestObjID = uint8(0); 
   Dx2edNearestObjIndex = uint8(0);
   Dx2edNearestObjID = uint8(0);
else
    Dx(MinIndex1st) = single(255);
    [MinDx2ed,MinIndex2ed] = min(Dx);
    Dx1stNearestObjIndex = uint8(MinIndex1st);
   Dx1stNearestObjID = uint8(ID(MinIndex1st)); 
   
   if (MinDx2ed > single(250))
     Dx2edNearestObjIndex = uint8(0);
     Dx2edNearestObjID = uint8(0);
   else
     Dx2edNearestObjIndex = uint8(MinIndex2ed);
     Dx2edNearestObjID = uint8(ID(MinIndex2ed));
   end
   

end
end

== stateflow chart PubIfDecisionTOS_MDL/TOS_20201112/TOS_2012080320/TOS/ACC/TOS_ACCLeftLane/ACCTargetPO24Infor/TOS_ACCPO2TargetInfor ==
  (default) -> (junction 1)
  (junction 1) -> (junction 3) [order 1] : [TOS_ACCPO2TargetIndex ~= uint8(0)]
  (junction 1) -> (junction 7) [order 2] : {TOS_ACCPO2TargetInfo.IDP2= uint8(0);
      | TOS_ACCPO2TargetInfo.dxP2=single(255);
      | TOS_ACCPO2TargetInfo.vxRelP2= single(0);
      | TOS_ACCPO2TargetInfo.axAbsGroundP2=single(0);
      | TOS_ACCPO2TargetInfo.rangeP2=single(0);
      | TOS_ACCPO2TargetInfo.targetExistP2= boolean(0);
      | TOS_ACCPO2TargetInfo.fu_typeP2= uint8(0);
      | TOS_ACCPO2TargetInfo.ObjMovingStateP2= uint8(0);
      | TOS_ACCPO2TargetInfo.ObjTypeP2= uint8(0);
      | TOS_ACCPO2TargetInfo.ObjDYP2=single(255);
      | TOS_ACCPO2TargetInfo.P2HeadingAngle=single(0);
      | TOS_ACCPO2TargetInfo.P2CutinProb= single(0);
      | }
  (junction 3) -> (junction 5) : {
      | TOS_ACCPO2TargetInfo.IDP2      =OFM_SignalVerification.Object_ID[TOS_ACCPO2TargetIndex- uint8(1)];
      | TOS_ACCPO2TargetInfo.dxP2      =OFM_SignalVerification.Object_DX[TOS_ACCPO2TargetIndex-uint8(1)];
      | TOS_ACCPO2TargetInfo.vxRelP2 =OFM_SignalVerification.Object_VX[TOS_ACCPO2TargetIndex-uint8(1)];
      |
      | TOS_ACCPO2TargetInfo.axAbsGroundP2      =TOS_AddAttributes.PP_axAbsGround[TOS_ACCPO2TargetIndex-uint8(1)];
      | TOS_ACCPO2TargetInfo.rangeP2                   =TOS_AddAttributes.PP_ObjToEgoCarFrontbump[TOS_ACCPO2TargetIndex-uint8(1)];
      | TOS_ACCPO2TargetInfo.targetExistP2           =boolean(1);
      | TOS_ACCPO2TargetInfo.fu_typeP2                =OFM_SignalVerification.Object_Fus_Type[TOS_ACCPO2TargetIndex-uint8(1)];
      | TOS_ACCPO2TargetInfo.ObjMovingStateP2  =TOS_AddAttributes.PP_MovingStateSignalProcessing[TOS_ACCPO2TargetIndex-uint8(1)];
      |
      | TOS_ACCPO2TargetInfo.ObjTypeP2           =OFM_SignalVerification.Object_Type[TOS_ACCPO2TargetIndex-uint8(1)];
      | TOS_ACCPO2TargetInfo.ObjDYP2              =OFM_SignalVerification.Object_DY[TOS_ACCPO2TargetIndex-uint8(1)];
      |
      | TOS_ACCPO2TargetInfo.P2HeadingAngle  =OFM_SignalVerification.Object_HeadingAngle[TOS_ACCPO2TargetIndex-uint8(1)];
      | TOS_ACCPO2TargetInfo.P2CutinProb         =TOS_ProbInLaneCalculat.PIL_CutinProb[TOS_ACCPO2TargetIndex-uint8(1)];
      | }
  (junction 5) -> (junction 7)
  (junction 7) -> (junction 11)
  data: OFM_SignalVerification input Bus: OFM_OBJ_BUS; TOS_AddAttributes input Bus: TOS_AddAttributes_BUS; TOS_ProbInLaneCalculat input Bus: PIL_ProbInLaneCalculat_BUS; TOS_ACCPO2TargetIndex input uint8; TOS_ACCPO2TargetInfo output Bus: TOS_ACCP2_BUS =0

== stateflow chart PubIfDecisionTOS_MDL/TOS_20201112/TOS_2012080320/TOS/ACC/TOS_ACCLeftLane/ACCTargetPO24Infor/TOS_ACCPO4TargetInfor ==
  (default) -> (junction 1)
  (junction 1) -> (junction 3) [order 1] : [TOS_ACCPO4TargetIndex ~= uint8(0)]
  (junction 1) -> (junction 7) [order 2] : {
      | TOS_ACCPO4TargetInfo.dyP4= uint8(0);
      | TOS_ACCPO4TargetInfo.dxP4=single(255);
      | TOS_ACCPO4TargetInfo.targetExistP4= boolean(1);
      | TOS_ACCPO4TargetInfo.ObjTypeP4= uint8(0);
      | }
  (junction 3) -> (junction 5) : {
      | TOS_ACCPO4TargetInfo.dyP4=OFM_SignalVerification.Object_DY[TOS_ACCPO4TargetIndex-uint8(1)];
      | TOS_ACCPO4TargetInfo.dxP4=OFM_SignalVerification.Object_DX[TOS_ACCPO4TargetIndex-uint8(1)];
      | TOS_ACCPO4TargetInfo.targetExistP4=boolean(1);
      | TOS_ACCPO4TargetInfo.ObjTypeP4=OFM_SignalVerification.Object_Type[TOS_ACCPO4TargetIndex-uint8(1)];
      | }
  (junction 5) -> (junction 7)
  (junction 7) -> (junction 11)
  data: OFM_SignalVerification input Bus: OFM_OBJ_BUS; TOS_AddAttributes input Bus: TOS_AddAttributes_BUS; TOS_ACCPO4TargetIndex input uint8; TOS_ACCPO4TargetInfo output Bus: TOS_ACCP4_BUS =0
